simulink model "dcMotorControl"  (R2014b)
settings: Solver=ode45  StartTime=0.0  StopTime=2  RelTol=1e-3
values from neighbouring files (symbols this model uses):
  Kd1 = 0    [plantDataAnalisys.m]
  Kd2 = 0    [plantDataAnalisys.m]
  Ki1 = 0    [plantDataAnalisys.m]
  Ki2 = 5    [plantDataAnalisys.m]
  Kp1 = 1000    [plantDataAnalisys.m]
  Kp2 = 5    [plantDataAnalisys.m]
  tfFirstVel = firstordertf(inputSignal(isInterval)',outputVel(isInterval)',time(isInterval)')    [plantDataAnalisys.m]
  tfSecondVel = secondordertf(inputSignal(isInterval)',outputVel(isInterval)',time(isInterval)')    [plantDataAnalisys.m]
settings Model: Creator=rafael  LastModifiedBy=rafael

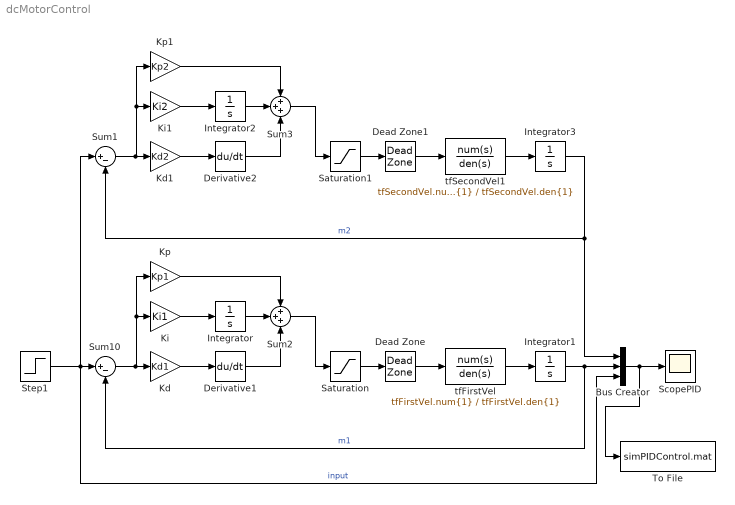
== system dcMotorControl ==
  Bus Creator : BusCreator  Inputs=3
  Dead Zone : DeadZone  LowerValue=deltaMinus  UpperValue=deltaPlus  SaturateOnIntegerOverflow=on
  Dead Zone1 : DeadZone  LowerValue=deltaMinus  UpperValue=deltaPlus  SaturateOnIntegerOverflow=on
  Derivative1 : Derivative
  Derivative2 : Derivative
  Integrator{,1..3} (4 alike) : Integrator
  Kd : Gain  Gain=Kd1
  Kd1 : Gain  Gain=Kd2
  Ki : Gain  Gain=Ki1
  Ki1 : Gain  Gain=Ki2
  Kp : Gain  Gain=Kp1
  Kp1 : Gain  Gain=Kp2
  Saturation : Saturate  UpperLimit=10  LowerLimit=-10
  Saturation1 : Saturate  UpperLimit=10  LowerLimit=-10
  ScopePID : Scope
      settings: ShowLegends=on  YMin=0  YMax=3
  Step1 : Step  SampleTime=0
  Sum1 : Sum  Inputs=|+-
  Sum10 : Sum  Inputs=|+-
  Sum2 : Sum  Inputs=+++
  Sum3 : Sum  Inputs=+++
  To File : ToFile  Filename=simPIDControl.mat  MatrixName=simData  SaveFormat=Timeseries
  tfFirstVel : TransferFcn  Numerator=tfFirstVel.num{1}  Denominator=tfFirstVel.den{1}
  tfSecondVel1 : TransferFcn  Numerator=tfSecondVel.num{1}  Denominator=tfSecondVel.den{1}
  wires:
  Sum10/1 -> Ki/1, Kp/1, Kd/1
  Sum2/1 -> Saturation/1
  Bus Creator/1 -> To File/1, ScopePID/1
  Saturation/1 -> Dead Zone/1
  Kp/1 -> Sum2/1
  Kd/1 -> Derivative1/1
  Ki/1 -> Integrator/1
  Integrator/1 -> Sum2/2
  Derivative1/1 -> Sum2/3
  tfFirstVel/1 -> Integrator1/1
  Integrator1/1 -> Sum10/2, Bus Creator/2  "m1"
  Dead Zone/1 -> tfFirstVel/1
  Step1/1 -> Sum1/1, Bus Creator/3, Sum10/1  "input"
  Sum1/1 -> Ki1/1, Kp1/1, Kd1/1
  Sum3/1 -> Saturation1/1
  Saturation1/1 -> Dead Zone1/1
  Kp1/1 -> Sum3/1
  Kd1/1 -> Derivative2/1
  Ki1/1 -> Integrator2/1
  Integrator2/1 -> Sum3/2
  Derivative2/1 -> Sum3/3
  tfSecondVel1/1 -> Integrator3/1
  Integrator3/1 -> Bus Creator/1, Sum1/2  "m2"
  Dead Zone1/1 -> tfSecondVel1/1
